simulink model "foc_controller"  (R2024b)
settings: Solver=FixedStepDiscrete  StartTime=0.0  StopTime=0.1  FixedStep=Ts  RelTol=1e-3
InitFcn:
  | cd(fileparts(which(bdroot)));
  | foc_params;
values from neighbouring files (symbols this model uses):
  duty_max = single(0.98)    [foc_params.m]
  duty_min = single(0.02)    [foc_params.m]
  Ki_d = single(Rs * wc)    [foc_params.m]
  Ki_q = single(Rs * wc)    [foc_params.m]
  Kp_d = single(Ld * wc)    [foc_params.m]
  Kp_q = single(Lq * wc)    [foc_params.m]
  Ts_ctrl = single(Ts)    [foc_params.m]
settings Model: Creator=Administrator  LastModifiedBy=Administrator
settings DataIOCC: SaveOutput=off  SaveTime=off  ReturnWorkspaceOutputs=off
settings OptimizationCC: DefaultParameterBehavior=Inlined  EnhancedBackFolding=on  PassReuseOutputArgsAs=Individual arguments  ZeroExternalMemoryAtStartup=off  ZeroInternalMemoryAtStartup=off  OptimizeBlockOrder=speed  DifferentSizesBufferReuse=on  OptimizationCustomize=off  EfficientTunableParamExpr=on
settings DebuggingCC: ParameterTunabilityLossMsg=error
settings HardwareCC: ProdBitPerPointer=32  ProdBitPerSizeT=32  ProdBitPerPtrDiffT=32  ProdLargestAtomicInteger=Long  ProdLargestAtomicFloat=Double  ProdWordSize=32  ProdHWDeviceType=ARM Compatible->ARM Cortex-M
settings SFSimCC: MATLABDynamicMemAlloc=off
settings RTWCC: Description=Embedded Coder  SystemTargetFile=ert.tlc  GenCodeOnly=on  TemplateMakefile=ert_default_tmf  GenerateReport=on
settings CodeAppCC: ForceParamTrailComments=on  IgnoreCustomStorageClasses=off  OperatorAnnotations=on  SimulinkDataObjDesc=on  SFDataObjDesc=on  InsertBlockDesc=on
settings ERTTargetCC: TargetLangStandard=C99 (ISO)  GenerateSampleERTMain=on  IncludeMdlTerminateFcn=off  SupportNonFinite=off  ERTCustomFileTemplate=example_file_process.tlc

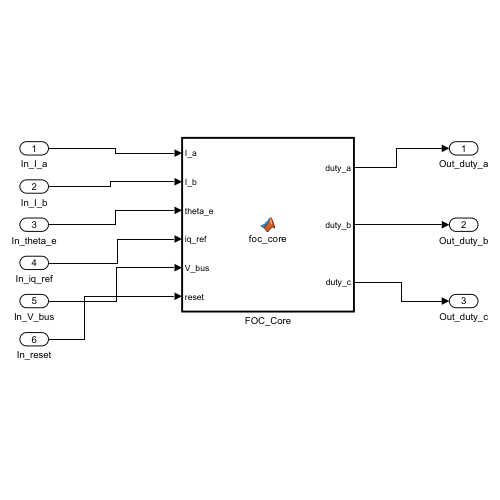
[thumbnail: Simulink's stored preview of the top-level diagram]
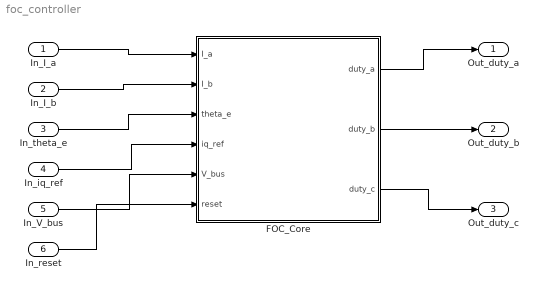
== system foc_controller ==
  In_I_a : Inport  OutDataTypeStr=single
  In_I_b : Inport  Port=2  OutDataTypeStr=single
  In_theta_e : Inport  Port=3  OutDataTypeStr=single
  In_iq_ref : Inport  Port=4  OutDataTypeStr=single
  In_V_bus : Inport  Port=5  OutDataTypeStr=single
  In_reset : Inport  Port=6  OutDataTypeStr=boolean
  FOC_Core : MATLAB Function  TreatAsAtomicUnit=on
  Out_duty_a : Outport  OutDataTypeStr=single
  Out_duty_b : Outport  Port=2  OutDataTypeStr=single
  Out_duty_c : Outport  Port=3  OutDataTypeStr=single
  wires:
  In_I_a/1 -> FOC_Core/1(I_a)
  In_I_b/1 -> FOC_Core/2(I_b)
  In_theta_e/1 -> FOC_Core/3(theta_e)
  In_iq_ref/1 -> FOC_Core/4(iq_ref)
  In_V_bus/1 -> FOC_Core/5(V_bus)
  FOC_Core/1(duty_a) -> Out_duty_a/1
  FOC_Core/2(duty_b) -> Out_duty_b/1
  FOC_Core/3(duty_c) -> Out_duty_c/1
  In_reset/1 -> FOC_Core/6(reset)

== matlab function foc_controller/FOC_Core ==
  data: I_a input single size=1; duty_a output single size=1; I_b input single size=1; theta_e input single size=1; iq_ref input single size=1; V_bus input single size=1; duty_b output single size=1; duty_c output single size=1; Ts_ctrl parameter single size=1; duty_min parameter single size=1; duty_max parameter single size=1; reset input boolean size=1; Kp_d parameter single size=1; Ki_d parameter single size=1; Kp_q parameter single size=1; Ki_q parameter single size=1
function [duty_a, duty_b, duty_c] = foc_core(I_a, I_b, theta_e, iq_ref, V_bus, Ts_ctrl, duty_min, duty_max, reset, Kp_d, Ki_d, Kp_q, Ki_q)
%#codegen
% FOC 电流环控制器 — 对齐固件 foc_interface.h
% Parameters (从 foc_params.m): Kp_d, Ki_d, Kp_q, Ki_q, Ts_ctrl, duty_min, duty_max

persistent int_d int_q
if isempty(int_d) || reset
    int_d = single(0);
    int_q = single(0);
end

id_ref = single(0);  % SPM: id=0 内部固定

% 1. IW 软件计算
I_c = -(I_a + I_b);

% 2. Clarke (等幅值 2/3)
ialpha = (2*I_a - I_b - I_c) / 3;
ibeta  = (sqrt(single(3)) * (I_b - I_c)) / 3;

% 3. Park
cos_e = cos(theta_e);
sin_e = sin(theta_e);
id_fb =  ialpha * cos_e + ibeta * sin_e;
iq_fb = -ialpha * sin_e + ibeta * cos_e;

% 4. PI (抗积分饱和)
V_lim = V_bus / sqrt(single(3));
err_d = id_ref - id_fb;
err_q = iq_ref - iq_fb;

vd_star = Kp_d * err_d + int_d;
vq_star = Kp_q * err_q + int_q;

v_mag = sqrt(vd_star*vd_star + vq_star*vq_star);
if v_mag > V_lim
    vd_star = vd_star * V_lim / v_mag;
    vq_star = vq_star * V_lim / v_mag;
else
    int_d = int_d + Ki_d * Ts_ctrl * err_d;
    int_q = int_q + Ki_q * Ts_ctrl * err_q;
end

% 5. 逆 Park
valpha = vd_star * cos_e - vq_star * sin_e;
vbeta  = vd_star * sin_e + vq_star * cos_e;

% 6. SVPWM (中性点注入)
va = valpha;
vb = -single(0.5)*valpha + (sqrt(single(3))/2)*vbeta;
vc = -single(0.5)*valpha - (sqrt(single(3))/2)*vbeta;
v_off = -(max(max(va,vb),vc) + min(min(va,vb),vc)) / 2;
va = va + v_off; vb = vb + v_off; vc = vc + v_off;

duty_a = max(duty_min, min(duty_max, va/V_bus + single(0.5)));
duty_b = max(duty_min, min(duty_max, vb/V_bus + single(0.5)));
duty_c = max(duty_min, min(duty_max, vc/V_bus + single(0.5)));
